simulink model "soc_WLAN_fpga"  (R2024b)
settings: Solver=FixedStepDiscrete  StartTime=0.0  StopTime=stopTime  RelTol=1e-3
PreLoadFcn:
  | addpath(fullfile(matlabroot,'toolbox','whdl','whdlexamples','whdlexamples'));
InitFcn:
  | addpath(fullfile(matlabroot,'toolbox','whdl','whdlexamples','whdlexamples'));
model workspace (MAT data in the model file):
  socvcb : containers.Map (value not decoded)
undefined symbols (not defined in the file): Add, bitRatePerOfdmSym, chanBW, coe, cpLen, dataUpsampleFactor, DelayValMaxNsdMinusLastPilotSc, DescramblerInitialSeed, designMultirateFIR, fftLen, filterLatency, filterUpsampleFactor, Fs, Hd, HT_MFMCS0, HT_MFMCS1, HT_MFMCS2, HT_MFMCS3, HT_MFMCS4, HT_MFMCS5, HT_MFMCS6, HT_MFMCS7, HTUnUsedScInd, inputSamplingRate, interp_coeff, maxPilotRefCounterVale, maxPilotsRef, maxPilotsRefNonHT, Ncol_HT, Ncol_NonHT, noDataSubCarriers, Non_HTMCS0, Non_HTMCS1, Non_HTMCS2, Non_HTMCS3, Non_HTMCS4, Non_HTMCS5, Non_HTMCS6, Non_HTMCS7, Nrow_HT, Nrow_NonHT, numDSC_HT, numDSC_HT_vhtSigB, numDSC_NonHT, numDscHT, numDscNonHT, numOfBitsPerOFDMSym, numOfDataBitsPerOFDMSym, numPilots, numScHT, numSCS_HT, numSCS_NonHT, pnSeq, QAM, rxDownsampleFactor, secondPIdx_HT, secondPIdx_NonHT, Shift, VHTMCS0, VHTMCS1 ... (+7)
libraries: hdlsllib x267, simulink x210, dspsigops x22, whdlutilities x10, whdlmod x9, dsphdlfiltering2 x5, dsphdlmathfun2 x4, whdledac x3, hwlogicconnlib x2, commhdlcrc x2, dsphdlsigops2 x2
(part 6 of 14)

== system soc_WLAN_fpga/WLAN/WLAN HDL/WLAN_Tx_Rx/WLAN_Rx/WLANHDLReceiver/DataRecovery/Deinterleaver/averageVhtSigBbits ==
  dataIn : Inport
  startIn : Inport  Port=2
  endIn : Inport  Port=3
  validIn : Inport  Port=4
  numSCSFlag : Inport  Port=5
  format : Inport  Port=6
  rst : Inport  Port=7
  Add : Sum
  Compare To Constant : simulink/Logic and Bit Operations/Compare To Constant  relop===  const=2  OutDataTypeStr=boolean
  Compare To Constant1 : simulink/Logic and Bit Operations/Compare To Constant  relop===  const=2  OutDataTypeStr=boolean
  Compare To Constant2 : simulink/Logic and Bit Operations/Compare To Constant  relop=<=  const=numDSC_HT-1  OutDataTypeStr=boolean
  Constant : Constant  Value=chanBW  OutDataTypeStr=fixdt(0,3,0)  SampleTime=-1
  Delay1 : Delay  DelayLength=54
  Delay2 : Delay  DelayLength=54
  Delay3 : Delay  DelayLength=54
  HDL Counter : hdlsllib/Sources/HDL Counter  CountType=Count limited  CountInit=0  CountStep=1  CountMax=65535  CountFromType=Initial value  CountFrom=0  CountResetPort=on  CountLoadPort=off  CountEnbPort=on  CountDirPort=off  CountHitOutputPort=off  CountDataType=Unsigned  CountWordLen=16  CountFracLen=0  CountSampTime=1
  Logical Operator : Logic  Inputs=4  AllPortsSameDT=off  OutDataTypeStr=boolean
  Logical Operator1 : Logic  AllPortsSameDT=off  OutDataTypeStr=boolean
  Shift Arithmetic : ArithShift  BitShiftNumber=1  BitShiftDirection=Right
  Switch : Switch  Criteria=u2 ~= 0  SaturateOnIntegerOverflow=off  InputSameDT=off
  Switch1 : Switch  Criteria=u2 ~= 0  SaturateOnIntegerOverflow=off  InputSameDT=off
  Switch2 : Switch  Criteria=u2 ~= 0  SaturateOnIntegerOverflow=off  InputSameDT=off
  dataOut : Outport
  startOut : Outport  Port=2
  endOut : Outport  Port=3
  validOut : Outport  Port=4
  wires:
  Constant/1 -> Compare To Constant/1
  Add/1 -> Shift Arithmetic/1
  numSCSFlag/1 -> Logical Operator/2
  dataIn/1 -> Add/1, Delay3/1, Switch/3
  Delay3/1 -> Add/2
  Compare To Constant/1 -> Logical Operator/1
  validIn/1 -> HDL Counter/2, Switch1/3, Delay1/1, Logical Operator1/2
  Delay1/1 -> Logical Operator1/1
  Logical Operator1/1 -> Switch1/1
  Logical Operator/1 -> Switch/2, Switch2/2, Switch1/2
  Switch1/1 -> validOut/1
  startIn/1 -> Switch2/3, Delay2/1
  Delay2/1 -> Switch2/1
  Switch2/1 -> startOut/1
  endIn/1 -> endOut/1
  Switch/1 -> dataOut/1
  Shift Arithmetic/1 -> Switch/1
  format/1 -> Compare To Constant1/1
  Compare To Constant1/1 -> Logical Operator/3
  HDL Counter/1 -> Compare To Constant2/1
  Compare To Constant2/1 -> Logical Operator/4
  rst/1 -> HDL Counter/1

== system soc_WLAN_fpga/WLAN/WLAN HDL/WLAN_Tx_Rx/WLAN_Rx/WLANHDLReceiver/FrameFormatDetectionAndSignalRecovery/CRCCheckAndBitInterpretation/numOFDMSymbolCalVHT ==
  note: Compute the number of OFDM data symbols for VHT frame format
  PSDULenNonHT : Inport
  numSTS : Inport  Port=2
  1-D Lookup Table : Lookup_n-D  NumberOfTableDimensions=1  BreakpointsForDimension1=[1:8]  IndexSearchMethod=Evenly spaced points  Table=9+[1 2 4 4 6 6 8 8]  ExtrapMethod=Clip  UseLastTableValue=on  InternalRulePriority=Speed  RndMeth=Simplest
  Add : Sum  Inputs=+-  OutDataTypeStr=uint16
  Delay : Delay  DelayLength=1
  Delay1 : Delay  DelayLength=1
  Delay2 : Delay  DelayLength=1
  Shift Arithmetic : ArithShift  BitShiftNumber=2  BitShiftDirection=Right
  rxTimeVHT : Subsystem
  numOFDMSymbVHT : Outport
  wires:
  numSTS/1 -> 1-D Lookup Table/1
  Shift Arithmetic/1 -> Delay/1
  1-D Lookup Table/1 -> Delay1/1
  Add/1 -> Delay2/1
  PSDULenNonHT/1 -> rxTimeVHT/1(In1)
  rxTimeVHT/1(Out1) -> Shift Arithmetic/1
  Delay/1 -> Add/1
  Delay1/1 -> Add/2
  Delay2/1 -> numOFDMSymbVHT/1

== system soc_WLAN_fpga/WLAN/WLAN HDL/WLAN_Tx_Rx/WLAN_Rx/WLANHDLReceiver/FrameFormatDetectionAndSignalRecovery/FormatIdentification/isQBPSK ==
  note: Threshold chose as half of used subcarriers in signal fields
  dataIn : Inport
  validIn : Inport  Port=2
  symbCount : Inport  Port=3
  rst : Inport  Port=4
  Compare To Constant : simulink/Logic and Bit Operations/Compare To Constant  relop===  const=5  OutDataTypeStr=boolean
  Compare To Constant1 : simulink/Logic and Bit Operations/Compare To Constant  relop===  const=6  OutDataTypeStr=boolean
  Complex to Real-Imag : ComplexToRealImag
  Constant : Constant  Value=48*0.5  OutDataTypeStr=fixdt(0,5,0)  SampleTime=-1
  Delay : Delay
  Delay1 : Delay
  Delay2 : Delay  DelayLength=1
  Delay3 : Delay  DelayLength=1
  Delay4 : Delay  DelayLength=3
  Delay5 : Delay  DelayLength=3
  Delay6 : Delay  DelayLength=3
  HDL Counter1 : hdlsllib/Sources/HDL Counter  CountType=Count limited  CountInit=0  CountStep=1  CountMax=256  CountFromType=Initial value  CountFrom=0  CountResetPort=on  CountLoadPort=off  CountEnbPort=on  CountDirPort=off  CountHitOutputPort=off  CountDataType=Unsigned  CountWordLen=9  CountFracLen=0  CountSampTime=1
  Logical Operator : Logic  AllPortsSameDT=off  OutDataTypeStr=boolean
  Logical Operator1 : Logic  AllPortsSameDT=off  OutDataTypeStr=boolean
  Logical Operator2 : Logic  Operator=OR  AllPortsSameDT=off  OutDataTypeStr=boolean
  Product : Product
  Product1 : Product
  Relational Operator : RelationalOperator  Operator=>  OutDataTypeStr=boolean  RndMeth=Simplest  InputSameDT=off
  Relational Operator1 : RelationalOperator  Operator=>  OutDataTypeStr=boolean  RndMeth=Simplest  InputSameDT=off
  To Workspace : ToWorkspace  VariableName=formatData  SampleTime=-1
      settings: Save2DSignal=2-D array (concatenate along first dimension)
  To Workspace1 : ToWorkspace  VariableName=formatValid  SampleTime=-1
      settings: Save2DSignal=2-D array (concatenate along first dimension)
  isQBPSK : Outport
  wires:
  Product/1 -> Delay2/1
  Complex to Real-Imag/2 -> Delay1/1
  Complex to Real-Imag/1 -> Delay/1
  Product1/1 -> Delay3/1
  dataIn/1 -> Delay5/1, Complex to Real-Imag/1
  HDL Counter1/1 -> Relational Operator1/1
  Constant/1 -> Relational Operator1/2
  Relational Operator1/1 -> isQBPSK/1
  Delay/1 -> Product/2, Product/1
  Delay1/1 -> Product1/2, Product1/1
  Delay2/1 -> Relational Operator/2
  Delay3/1 -> Relational Operator/1
  Relational Operator/1 -> Logical Operator/1
  Logical Operator/1 -> HDL Counter1/2
  validIn/1 -> Delay4/1
  Delay4/1 -> Logical Operator1/1
  symbCount/1 -> Compare To Constant1/1, Compare To Constant/1
  Compare To Constant/1 -> Logical Operator2/1
  Logical Operator1/1 -> Logical Operator/2, To Workspace1/1
  Delay6/1 -> Logical Operator1/2
  Compare To Constant1/1 -> Logical Operator2/2
  Logical Operator2/1 -> Delay6/1
  rst/1 -> HDL Counter1/1
  Delay5/1 -> To Workspace/1

== system soc_WLAN_fpga/WLAN/WLAN HDL/WLAN_Tx_Rx/WLAN_Rx/WLANHDLReceiver/FrameFormatDetectionAndSignalRecovery/SignalBitRecovery/Deinterleaver Block ==
  note: Give null output if valid is LOW
  dataIn : Inport
  startIn : Inport  Port=2
  endIn : Inport  Port=3
  validIn : Inport  Port=4
  Constant : Constant  Value=0  OutDataTypeStr=Inherit: Inherit via back propagation  SampleTime=-1
  Delay{1,3..6,9..11} (8 alike) : Delay  DelayLength=1
  Delay12 : Delay  DelayLength=7
  Delay13 : Delay  DelayLength=7
  Delay14 : Delay  DelayLength=7
  Delay{2,15..17} (4 alike) : Delay
  Delay7 : Delay  DelayLength=1  InitialCondition=true
  Delay8 : Delay  DelayLength=1  InitialCondition=true
  Generate Ready : Subsystem
  Logical Operator : Logic  IconShape=distinctive  AllPortsSameDT=off  OutDataTypeStr=boolean
  RAM : hdlsllib/HDL RAMs/Simple Dual Port RAM  ram_size=nextpow2(2*maxBlkSize)
  Read Logic : Subsystem
  Store Block Lengths : hdlsllib/HDL RAMs/HDL FIFO  fifo_size=4  mode=Classic  ratio=1  push_msg=Warning  pop_msg=Ignore  show_empty=off  show_full=off  show_num=on  LabelModeActiveChoice_Mode=Classic  rst_port=off
  Switch : Switch  Criteria=u2 ~= 0  SaturateOnIntegerOverflow=off
  Write Logic : Subsystem
  dataOut : Outport
  startOut : Outport  Port=2
  endOut : Outport  Port=3
  validOut : Outport  Port=4
  ready : Outport  Port=5
  wires:
  Delay17/1 -> Delay14/1
  Delay16/1 -> Delay12/1
  Delay15/1 -> Delay13/1
  Delay14/1 -> RAM/1
  Delay12/1 -> RAM/2
  Delay13/1 -> RAM/3
  Constant/1 -> Switch/3
  Switch/1 -> dataOut/1
  RAM/1 -> Switch/1
  Generate Ready/1(ready) -> ready/1, [ready]
  Read Logic/6(advPop) -> Generate Ready/1(advPop)
  Write Logic/5(endReady) -> Generate Ready/4(endReady)
  Delay7/1 -> Logical Operator/2
  validIn/1 -> Logical Operator/1
  Logical Operator/1 -> Write Logic/2(valid)
  [ready] -> Delay7/1
  Read Logic/5(pop) -> [b]
  Delay6/1 -> startOut/1
  Delay10/1 -> validOut/1, Switch/2
  Delay5/1 -> endOut/1
  Delay11/1 -> Store Block Lengths/2
  Delay9/1 -> Store Block Lengths/1
  Delay4/1 -> Delay15/1
  Delay3/1 -> Delay16/1
  Delay1/1 -> Delay17/1
  Delay8/1 -> Store Block Lengths/3, Generate Ready/3(pop)
  [b] -> Delay8/1
  Read Logic/3(end) -> Delay5/1
  Read Logic/2(start) -> Delay6/1
  Read Logic/1(rdAddr) -> RAM/4
  Store Block Lengths/1 -> Read Logic/1(fifoData)
  Read Logic/4(valid) -> Delay10/1
  Write Logic/4(endOut) -> Delay11/1
  Write Logic/3(count) -> Delay9/1
  Write Logic/2(wrValid) -> Delay4/1
  Write Logic/1(wrAddr) -> Delay3/1
  endIn/1 -> Write Logic/3(end)
  startIn/1 -> Write Logic/1(start)
  Delay2/1 -> Delay1/1
  dataIn/1 -> Delay2/1
  Store Block Lengths/2 -> Read Logic/2(fifoCount), Generate Ready/2(fifoCount)

== system soc_WLAN_fpga/WLAN/WLAN HDL/WLAN_Tx_Rx/WLAN_Rx/WLANHDLReceiver/FrameFormatDetectionAndSignalRecovery/SignalBitRecovery/ViterbiDecoder ==
  llr : Inport
  ctrlIn : Inport  Port=2
  Gain : Gain  Gain=-1  OutDataTypeStr=Inherit: Same as input
  Viterbi Decoder : whdledac/Viterbi Decoder  ConstraintLength=7  CodeGenerator=[133 171]  ErasureInputPort=off  Tbd=32  TerminationMethod=Truncated  ResetInputPort=off  SimulateUsing=Code generation
  bit : Outport
  ctrlOut : Outport  Port=2
  wires:
  Viterbi Decoder/1 -> bit/1
  Viterbi Decoder/2 -> ctrlOut/1
  ctrlIn/1 -> Viterbi Decoder/2
  llr/1 -> Gain/1
  Gain/1 -> Viterbi Decoder/1

== system soc_WLAN_fpga/WLAN/WLAN HDL/WLAN_Tx_Rx/WLAN_Rx/WLANHDLReceiver/FrameFormatDetectionAndSignalRecovery/averageSigFieldsFor40MHz/averager ==
  In1 : Inport
  enb : Inport  Port=2
  rst : Inport  Port=3
  Add : Sum
  Compare To Constant : simulink/Logic and Bit Operations/Compare To Constant  relop=>=  const=numDSC_NonHT/2  OutDataTypeStr=boolean
  Constant : Constant  Value=complex(0,0)  OutDataTypeStr=Inherit: Inherit via back propagation  SampleTime=-1
  Delay : Delay  DelayLength=fftLen/2
  Gain : Gain  Gain=0.5
  HDL Counter : hdlsllib/Sources/HDL Counter  CountType=Count limited  CountInit=0  CountStep=1  CountMax=numDSC_NonHT-1  CountFromType=Initial value  CountFrom=0  CountResetPort=on  CountLoadPort=off  CountEnbPort=on  CountDirPort=off  CountHitOutputPort=off  CountDataType=Unsigned  CountWordLen=8  CountFracLen=0  CountSampTime=1
  Logical Operator : Logic  AllPortsSameDT=off  OutDataTypeStr=boolean
  Switch : Switch  Criteria=u2 ~= 0  SaturateOnIntegerOverflow=off  InputSameDT=off
  Out1 : Outport
  validIn : Outport  Port=2
  wires:
  Constant/1 -> Switch/3
  In1/1 -> Delay/1, Add/1
  HDL Counter/1 -> Compare To Constant/1
  Delay/1 -> Add/2
  Compare To Constant/1 -> Logical Operator/1, Switch/2
  Add/1 -> Gain/1
  enb/1 -> Logical Operator/2, HDL Counter/2
  Switch/1 -> Out1/1
  Gain/1 -> Switch/1
  Logical Operator/1 -> validIn/1
  rst/1 -> HDL Counter/1

== system soc_WLAN_fpga/WLAN/WLAN HDL/WLAN_Tx_Rx/WLAN_Rx/WLANHDLReceiver/HT_VHTCPEEstAndCorrection/CPECorrector/Reciprocal ==
  dataIn : Inport
  Compare To Constant : simulink/Logic and Bit Operations/Compare To Constant  relop=<  const=0  OutDataTypeStr=boolean
  Data Type Conversion : DataTypeConversion  OutDataTypeStr=fixdt(1,WL,0)  ConvertRealWorld=Stored Integer (SI)  SaturateOnIntegerOverflow=off  RndMeth=Floor
  Data Type Conversion1 : DataTypeConversion  OutDataTypeStr=fixdt(0,LUTAddrWL,0)  ConvertRealWorld=Stored Integer (SI)  SaturateOnIntegerOverflow=off  RndMeth=Floor
  Data Type Conversion2 : DataTypeConversion  OutDataTypeStr=fixdt(0,WL-LUTAddrWL,0)  ConvertRealWorld=Stored Integer (SI)  SaturateOnIntegerOverflow=off  RndMeth=Floor
  Delay : Delay  DelayLength=1
  Delay1 : Delay  DelayLength=1
  Delay2 : Delay  DelayLength=1
  Extract Bits : simulink/Logic and Bit Operations/Extract Bits  bitsToExtract=Range ending with least significant bit  numBits=LUTAddrWL  bitIdxRange=[0 7]  outScalingMode=Treat bit field as an integer
  Function Impl : Subsystem
  dataOut : Outport
  wires:
  Data Type Conversion2/1 -> Function Impl/1(switch)
  Delay2/1 -> Data Type Conversion1/1
  Delay1/1 -> Data Type Conversion2/1
  Delay/1 -> Extract Bits/1, Compare To Constant/1
  Function Impl/1(functionValues) -> dataOut/1
  Data Type Conversion1/1 -> Function Impl/2(LUTAddr)
  Compare To Constant/1 -> Delay1/1
  Data Type Conversion/1 -> Delay/1
  Extract Bits/1 -> Delay2/1
  dataIn/1 -> Data Type Conversion/1

== system soc_WLAN_fpga/WLAN/WLAN HDL/WLAN_Tx_Rx/WLAN_Rx/WLANHDLReceiver/HT_VHTCPEEstAndCorrection/CPEEstimator/RefrenceSignalGen ==
  note: reference pilots are stored in LUT for 4 symbols
      | pilots for 4 symbols are stored to avoid modulo operation
  note: Counter for pilot Subcarriers for 4 Symbols
  loadIn : Inport
  vhtSigB : Inport  Port=2
  rst : Inport  Port=3
  1-D Lookup Table1 : Lookup_n-D  NumberOfTableDimensions=1  BreakpointsForDimension1=[0:maxPilotsRef^2-1]  IndexSearchMethod=Evenly spaced points  Table=PilotsDataDec.'  ExtrapMethod=Clip  UseLastTableValue=on  InternalRulePriority=Speed  OutDataTypeStr=fixdt(1,2,0)  RndMeth=Simplest
  Compare To Constant : simulink/Logic and Bit Operations/Compare To Constant  relop===  const=numSCS_HT-1  OutDataTypeStr=boolean
  Delay : Delay  DelayLength=1  InitialCondition=0  UseCircularBuffer=on
  HDL Counter : hdlsllib/Sources/HDL Counter  CountType=Count limited  CountInit=0  CountStep=1  CountMax=maxPilotsRef^2-1  CountFromType=Initial value  CountFrom=0  CountResetPort=on  CountLoadPort=off  CountEnbPort=on  CountDirPort=off  CountHitOutputPort=off  CountDataType=Unsigned  CountWordLen=maxPilotRefCounterVale*2  CountFracLen=0  CountSampTime=1
  HDL Counter1 : hdlsllib/Sources/HDL Counter  CountType=Count limited  CountInit=0  CountStep=1  CountMax=numSCS_HT-1  CountFromType=Initial value  CountFrom=0  CountResetPort=on  CountLoadPort=off  CountEnbPort=on  CountDirPort=off  CountHitOutputPort=off  CountDataType=Unsigned  CountWordLen=8  CountFracLen=0  CountSampTime=1
  Logical Operator : Logic  AllPortsSameDT=off  OutDataTypeStr=boolean
  Logical Operator1 : Logic  Operator=OR  AllPortsSameDT=off  OutDataTypeStr=boolean
  RefPilotsOut : Outport
  wires:
  HDL Counter/1 -> 1-D Lookup Table1/1
  1-D Lookup Table1/1 -> Delay/1
  loadIn/1 -> HDL Counter/2
  vhtSigB/1 -> Logical Operator/2, HDL Counter1/2
  HDL Counter1/1 -> Compare To Constant/1
  Compare To Constant/1 -> Logical Operator/1
  Logical Operator/1 -> Logical Operator1/1
  rst/1 -> Logical Operator1/2, HDL Counter1/1
  Logical Operator1/1 -> HDL Counter/1
  Delay/1 -> RefPilotsOut/1

== system soc_WLAN_fpga/WLAN/WLAN HDL/WLAN_Tx_Rx/WLAN_Rx/WLANHDLReceiver/HT_VHTChannelEstAndEqualize/ChannelEqualizer/validForEqualization ==
  note: selecting Data field for equalization
  validIn : Inport
  symbNum : Inport  Port=2
  rst : Inport  Port=3
  Compare To Constant1 : simulink/Logic and Bit Operations/Compare To Constant  relop=>=  const=9  OutDataTypeStr=boolean
  Compare To Constant2 : simulink/Logic and Bit Operations/Compare To Constant  relop===  const=9  OutDataTypeStr=boolean
  Compare To Constant3 : simulink/Logic and Bit Operations/Compare To Constant  relop===  const=0  OutDataTypeStr=boolean
  HDL Counter : hdlsllib/Sources/HDL Counter  CountType=Count limited  CountInit=0  CountStep=1  CountMax=numSCS_HT-1  CountFromType=Initial value  CountFrom=0  CountResetPort=on  CountLoadPort=off  CountEnbPort=on  CountDirPort=off  CountHitOutputPort=off  CountDataType=Unsigned  CountWordLen=8  CountFracLen=0  CountSampTime=1
  Logical Operator : Logic  AllPortsSameDT=off  OutDataTypeStr=boolean
  Logical Operator1 : Logic  AllPortsSameDT=off  OutDataTypeStr=boolean
  Logical Operator2 : Logic  AllPortsSameDT=off  OutDataTypeStr=boolean
  hValid : Outport
  DataValid : Outport  Port=2
  loadH : Outport  Port=3
  wires:
  validIn/1 -> Logical Operator1/1, Logical Operator/1
  Logical Operator/1 -> DataValid/1
  symbNum/1 -> Compare To Constant2/1, Compare To Constant1/1
  Compare To Constant1/1 -> Logical Operator/2
  Compare To Constant2/1 -> Logical Operator1/2
  Logical Operator2/1 -> loadH/1
  HDL Counter/1 -> Compare To Constant3/1
  Logical Operator1/1 -> Logical Operator2/2, HDL Counter/2, hValid/1
  Compare To Constant3/1 -> Logical Operator2/1
  rst/1 -> HDL Counter/1

== system soc_WLAN_fpga/WLAN/WLAN HDL/WLAN_Tx_Rx/WLAN_Rx/WLANHDLReceiver/NonHTCPEEstAndCorrection/CPECorrector/Reciprocal ==
  dataIn : Inport
  Compare To Constant : simulink/Logic and Bit Operations/Compare To Constant  relop=<  const=0  OutDataTypeStr=boolean
  Data Type Conversion : DataTypeConversion  OutDataTypeStr=fixdt(1,WL,0)  ConvertRealWorld=Stored Integer (SI)  SaturateOnIntegerOverflow=off  RndMeth=Floor
  Data Type Conversion1 : DataTypeConversion  OutDataTypeStr=fixdt(0,LUTAddrWL,0)  ConvertRealWorld=Stored Integer (SI)  SaturateOnIntegerOverflow=off  RndMeth=Floor
  Data Type Conversion2 : DataTypeConversion  OutDataTypeStr=fixdt(0,WL-LUTAddrWL,0)  ConvertRealWorld=Stored Integer (SI)  SaturateOnIntegerOverflow=off  RndMeth=Floor
  Delay : Delay  DelayLength=1
  Delay1 : Delay  DelayLength=1
  Delay2 : Delay  DelayLength=1
  Extract Bits : simulink/Logic and Bit Operations/Extract Bits  bitsToExtract=Range ending with least significant bit  numBits=LUTAddrWL  bitIdxRange=[0 7]  outScalingMode=Treat bit field as an integer
  Function Impl : Subsystem
  dataOut : Outport
  wires:
  Data Type Conversion2/1 -> Function Impl/1(switch)
  Delay2/1 -> Data Type Conversion1/1
  Delay1/1 -> Data Type Conversion2/1
  Delay/1 -> Extract Bits/1, Compare To Constant/1
  Function Impl/1(functionValues) -> dataOut/1
  Data Type Conversion1/1 -> Function Impl/2(LUTAddr)
  Compare To Constant/1 -> Delay1/1
  Data Type Conversion/1 -> Delay/1
  Extract Bits/1 -> Delay2/1
  dataIn/1 -> Data Type Conversion/1

== system soc_WLAN_fpga/WLAN/WLAN HDL/WLAN_Tx_Rx/WLAN_Rx/WLANHDLReceiver/NonHTCPEEstAndCorrection/CPEEstimator/RefrenceSignalGen ==
  note: reference pilots are stored in LUT for 4 symbols
      | pilots for 4 symbols are stored to avoid modulo operation
  note: Counter for pilot Subcarriers for 4 Symbols
  loadIn : Inport
  rst : Inport  Port=2
  1-D Lookup Table1 : Lookup_n-D  NumberOfTableDimensions=1  BreakpointsForDimension1=[0:maxPilotsRefNonHT-1]  IndexSearchMethod=Evenly spaced points  Table=PilotLUTSignalNonHT.'  TableDataTypeStr=fixdt(1,2,0)  ExtrapMethod=Clip  UseLastTableValue=on  InternalRulePriority=Speed  OutDataTypeStr=fixdt(1,2,0)  RndMeth=Simplest
  Delay2 : Delay  DelayLength=1  InitialCondition=0  UseCircularBuffer=on
  HDL Counter : hdlsllib/Sources/HDL Counter  CountType=Count limited  CountInit=0  CountStep=1  CountMax=maxPilotsRefNonHT-1  CountFromType=Initial value  CountFrom=0  CountResetPort=on  CountLoadPort=off  CountEnbPort=on  CountDirPort=off  CountHitOutputPort=off  CountDataType=Unsigned  CountWordLen=3  CountFracLen=0  CountSampTime=1
  RefPilotsOut : Outport
  wires:
  HDL Counter/1 -> 1-D Lookup Table1/1
  1-D Lookup Table1/1 -> Delay2/1
  loadIn/1 -> HDL Counter/2
  rst/1 -> HDL Counter/1
  Delay2/1 -> RefPilotsOut/1

== system soc_WLAN_fpga/WLAN/WLAN HDL/WLAN_Tx_Rx/WLAN_Rx/WLANHDLReceiver/NonHTChannelEstAndEqualize/ChannelEqualizer/NonHTDataSelector ==
  note: selecting from L-SIG field to L-Data for equalization
  validIn : Inport
  symbNum : Inport  Port=2
  Compare To Constant1 : simulink/Logic and Bit Operations/Compare To Constant  relop=>=  const=4  OutDataTypeStr=boolean
  Logical Operator : Logic  AllPortsSameDT=off  OutDataTypeStr=boolean
  NonHTValid : Outport
  wires:
  validIn/1 -> Logical Operator/2
  Logical Operator/1 -> NonHTValid/1
  symbNum/1 -> Compare To Constant1/1
  Compare To Constant1/1 -> Logical Operator/1

== system soc_WLAN_fpga/WLAN/WLAN HDL/WLAN_Tx_Rx/WLAN_Rx/WLANHDLReceiver/OFDMDemodulation/Symbol Counter/vhtRotation ==
  u : Inport
  In2 : Inport  Port=2
  Compare To Constant : simulink/Logic and Bit Operations/Compare To Constant  relop=>=  const=fftLen/2  OutDataTypeStr=boolean
  Constant : Constant  Value=fi(1/1i,1,2,0)  SampleTime=-1
  Product : Product
  Switch : Switch  Criteria=u2 ~= 0  SaturateOnIntegerOverflow=off  InputSameDT=off
  dataOut : Outport
  wires:
  In2/1 -> Switch/3, Product/1
  Constant/1 -> Product/2
  Switch/1 -> dataOut/1
  Compare To Constant/1 -> Switch/2
  u/1 -> Compare To Constant/1
  Product/1 -> Switch/1

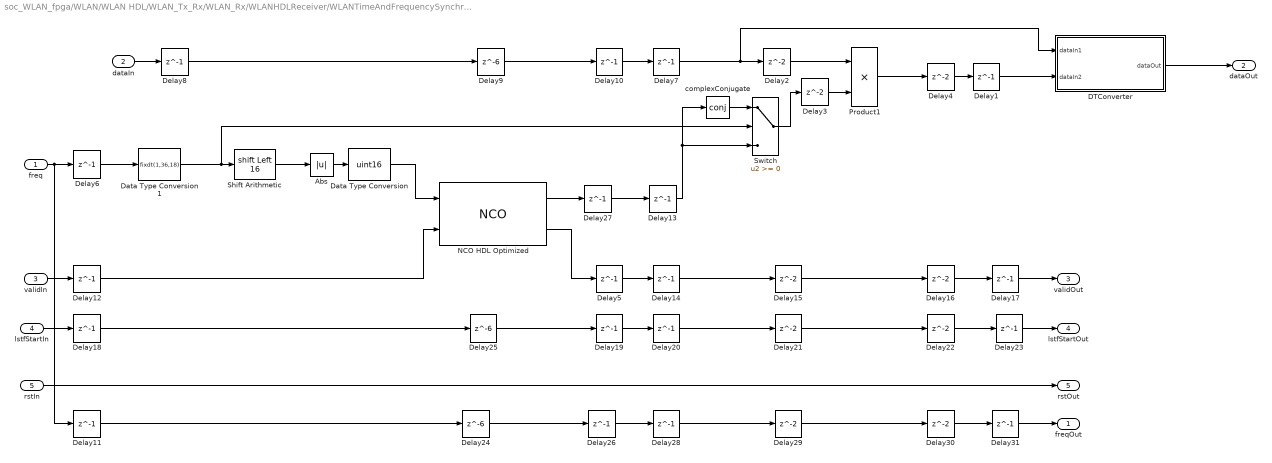
== system soc_WLAN_fpga/WLAN/WLAN HDL/WLAN_Tx_Rx/WLAN_Rx/WLANHDLReceiver/WLANTimeAndFrequencySynchronization/Coarse CFO Estimation and Correction/Coarse CFO Correction ==
  freq : Inport
  dataIn : Inport  Port=2
  validIn : Inport  Port=3
  lstfStartIn : Inport  Port=4
  rstIn : Inport  Port=5
  Abs : Abs  SaturateOnIntegerOverflow=off
  DTConverter : MATLAB Function  TreatAsAtomicUnit=on
  Data Type Conversion : DataTypeConversion  OutDataTypeStr=uint16  RndMeth=Round  SaturateOnIntegerOverflow=off
  Data Type Conversion1 : DataTypeConversion  OutDataTypeStr=fixdt(1,36,18)  SaturateOnIntegerOverflow=off  RndMeth=Floor
  Delay{1,5..8,10..14,17..20,23,26..28,31} (19 alike) : Delay  DelayLength=1  InitialCondition=0  UseCircularBuffer=on
  Delay{2..4,15..16,21..22,29..30} (9 alike) : Delay  InitialCondition=0  UseCircularBuffer=on
  Delay24 : Delay  DelayLength=6  InitialCondition=0  UseCircularBuffer=on
  Delay25 : Delay  DelayLength=6  InitialCondition=0  UseCircularBuffer=on
  Delay9 : Delay  DelayLength=6  InitialCondition=0  UseCircularBuffer=on
  NCO HDL Optimized : dsphdlsigops2/NCO  PhaseIncrementSource=Input port  PhaseIncrement=100  PhaseOffsetSource=Property  PhaseOffset=0  DitherSource=None  NumDitherBits=4  SamplesPerFrame=1  LUTCompress=off  ResetAction=off  Waveform=Complex exponential  PhasePort=off  SimulateUsing=Code generation  AccumulatorWL=16  PhaseQuantization=on  NumQuantizerAccumulatorBits=16  OutputDataType=Binary point scaling  OutputWL=16  OutputFL=14
  Product1 : Product
  Shift Arithmetic : ArithShift  BitShiftNumber=16  BitShiftDirection=Left
  Switch : Switch  SaturateOnIntegerOverflow=off  InputSameDT=off
  complexConjugate : Math  Operator=conj  SignedPower=on
  freqOut : Outport  VectorParamsAs1DForOutWhenUnconnected=off
  dataOut : Outport  Port=2  VectorParamsAs1DForOutWhenUnconnected=off
  validOut : Outport  Port=3  VectorParamsAs1DForOutWhenUnconnected=off
  lstfStartOut : Outport  Port=4  VectorParamsAs1DForOutWhenUnconnected=off
  rstOut : Outport  Port=5  VectorParamsAs1DForOutWhenUnconnected=off
  wires:
  Delay25/1 -> Delay19/1
  NCO HDL Optimized/2 -> Delay5/1
  Delay9/1 -> Delay10/1
  Delay23/1 -> lstfStartOut/1
  Delay22/1 -> Delay23/1
  Delay21/1 -> Delay22/1
  Delay20/1 -> Delay21/1
  Delay19/1 -> Delay20/1
  Delay18/1 -> Delay25/1
  lstfStartIn/1 -> Delay18/1
  Delay5/1 -> Delay14/1
  freq/1 -> Delay11/1, Delay6/1
  Delay4/1 -> Delay1/1
  dataIn/1 -> Delay8/1
  Delay17/1 -> validOut/1
  Delay3/1 -> Product1/2
  Delay16/1 -> Delay17/1
  validIn/1 -> Delay12/1
  Delay10/1 -> Delay7/1
  Delay15/1 -> Delay16/1
  Delay2/1 -> Product1/1
  Product1/1 -> Delay4/1
  Delay13/1 -> complexConjugate/1, Switch/3
  Delay8/1 -> Delay9/1
  Delay7/1 -> DTConverter/1(dataIn1), Delay2/1
  Delay14/1 -> Delay15/1
  Delay27/1 -> Delay13/1
  Data Type Conversion/1 -> NCO HDL Optimized/1
  Delay12/1 -> NCO HDL Optimized/2
  NCO HDL Optimized/1 -> Delay27/1
  rstIn/1 -> rstOut/1
  Delay6/1 -> Data Type Conversion1/1
  Data Type Conversion1/1 -> Shift Arithmetic/1, Switch/2
  DTConverter/1(dataOut) -> dataOut/1
  Delay1/1 -> DTConverter/2(dataIn2)
  complexConjugate/1 -> Switch/1
  Switch/1 -> Delay3/1
  Shift Arithmetic/1 -> Abs/1
  Abs/1 -> Data Type Conversion/1
  Delay11/1 -> Delay24/1
  Delay24/1 -> Delay26/1
  Delay26/1 -> Delay28/1
  Delay28/1 -> Delay29/1
  Delay29/1 -> Delay30/1
  Delay30/1 -> Delay31/1
  Delay31/1 -> freqOut/1

== system soc_WLAN_fpga/WLAN/WLAN HDL/WLAN_Tx_Rx/WLAN_Rx/WLANHDLReceiver/WLANTimeAndFrequencySynchronization/Coarse CFO Estimation and Correction/Coarse CFO Estimation ==
  dataIn : Inport
  validIn : Inport  Port=2
  LSTF_start : Inport  Port=3
  rstIn : Inport  Port=4
  Complex to Magnitude-Angle HDL Optimized : dsphdlmathfun2/Complex to Magnitude-Angle  NumIterationsSource=Auto  NumIterations=30  OutputFormat=Angle  AngleFormat=Normalized  ScaleOutput=off  ScalingMethod=Shift-Add  SimulateUsing=Code generation
  Delay10 : Delay  DelayLength=wlanConfig.lstfLen  InitialCondition=0
  Delay{11,13,16..17,21} (5 alike) : Delay  DelayLength=1  InitialCondition=0  UseCircularBuffer=on
  Delay14 : Delay  DelayLength=wlanConfig.lstfLen  InitialCondition=0
  Delay15 : Delay  InitialCondition=0  UseCircularBuffer=on
  Delay22 : Delay  DelayLength=35  InitialCondition=0  UseCircularBuffer=on
  Delay23 : Delay  DelayLength=round(wlanConfig.lstfLen*0.75)+8*wlanConfig.lstfLen-1  InitialCondition=0  UseCircularBuffer=on
  Delay{24..27} (4 alike) : Delay  DelayLength=1
  Delay4 : Delay  DelayLength=35  InitialCondition=0  UseCircularBuffer=on
  Delay5 : Delay  DelayLength=35  InitialCondition=0  UseCircularBuffer=on
  Delay6 : Delay  InitialCondition=0  UseCircularBuffer=on
  Delay7 : Delay  DelayLength=round(wlanConfig.lstfLen*0.75)+8*wlanConfig.lstfLen-1  InitialCondition=0  UseCircularBuffer=on
  Delay9 : Delay  DelayLength=round(wlanConfig.lstfLen*0.75)+8*wlanConfig.lstfLen-1  InitialCondition=0  UseCircularBuffer=on
  Shift Arithmetic : ArithShift  BitShiftNumber=log2(2*wlanConfig.lstfLen)  BitShiftDirection=Right
  Unit Delay Enabled Resettable Synchronous : hdlsllib/Discrete/Unit Delay Enabled Resettable Synchronous  InitialCondition=0.0  SampleTime=-1
  averager : Subsystem
  correlator : Subsystem
  Freq : Outport  VectorParamsAs1DForOutWhenUnconnected=off
  dataOut : Outport  Port=2  VectorParamsAs1DForOutWhenUnconnected=off
  validData : Outport  Port=3  VectorParamsAs1DForOutWhenUnconnected=off
  lstfStart : Outport  Port=4  VectorParamsAs1DForOutWhenUnconnected=off
  rstOut : Outport  Port=5  VectorParamsAs1DForOutWhenUnconnected=off
  wires:
  validIn/1 -> Delay10/1
  dataIn/1 -> Delay14/1, correlator/1(dataIn)
  LSTF_start/1 -> correlator/2(lstf_start)
  Delay9/1 -> Delay5/1
  Complex to Magnitude-Angle HDL Optimized/2 -> Delay13/1
  Delay5/1 -> Delay16/1
  Delay4/1 -> Delay17/1
  Complex to Magnitude-Angle HDL Optimized/1 -> Delay11/1
  Delay16/1 -> validData/1
  Delay17/1 -> dataOut/1
  Delay10/1 -> Delay6/1
  Delay6/1 -> Delay26/1
  Delay11/1 -> Shift Arithmetic/1
  Delay7/1 -> Delay4/1
  Delay26/1 -> Delay9/1
  Delay14/1 -> Delay15/1
  Delay15/1 -> Delay27/1
  Delay27/1 -> Delay7/1
  Delay22/1 -> Delay21/1
  correlator/2(load) -> Delay25/1
  Delay23/1 -> Delay22/1
  Delay21/1 -> lstfStart/1
  Delay25/1 -> Delay23/1, averager/2(load)
  Shift Arithmetic/1 -> Unit Delay Enabled Resettable Synchronous/1
  Unit Delay Enabled Resettable Synchronous/1 -> Freq/1
  Delay13/1 -> Unit Delay Enabled Resettable Synchronous/2
  rstIn/1 -> averager/3(rst), Unit Delay Enabled Resettable Synchronous/3, rstOut/1
  correlator/1(corrOut) -> Delay24/1
  averager/1(avgCorr) -> Complex to Magnitude-Angle HDL Optimized/1
  averager/2(validOut) -> Complex to Magnitude-Angle HDL Optimized/2
  Delay24/1 -> averager/1(corrIn)

== system soc_WLAN_fpga/WLAN/WLAN HDL/WLAN_Tx_Rx/WLAN_Rx/WLANHDLReceiver/WLANTimeAndFrequencySynchronization/Coarse Time Sync/correlator ==
  dataIn : Inport
  validIn : Inport  Port=2
  startIn : Inport  Port=3
  Constant : Constant  Value=complex(0,0)  VectorParams1D=off  OutDataTypeStr=Inherit: Inherit via back propagation  SampleTime=-1
  Delay : Delay
  Delay1 : Delay  DelayLength=1
  Delay2 : Delay  DelayLength=wlanConfig.lstfLen-1
  Delay3 : Delay
  Delay4 : Delay  DelayLength=1
  Delay5 : Delay  DelayLength=1
  Logical Operator : Logic  AllPortsSameDT=off  OutDataTypeStr=boolean
  MagnitudeSquared : Subsystem
  MovingSum : Subsystem  InitFcn=Simulink.suppressDiagnostic(gcb, 'SimulinkFixedPoint:util:Overflowoccurred');
  Shift Arithmetic : ArithShift  BitShiftNumber=log2(wlanConfig.lstfLen)  BitShiftDirection=Right
  Switch : Switch  Criteria=u2 > Threshold  SaturateOnIntegerOverflow=off  InputSameDT=off
  delayedCorrelation : Subsystem
  dataOut : Outport
  validOut : Outport  Port=2
  wires:
  MagnitudeSquared/2(validOut) -> Delay3/1
  MovingSum/2(validOut) -> Delay2/1, Logical Operator/2
  Switch/1 -> Shift Arithmetic/1
  Constant/1 -> Switch/3
  MovingSum/1(dataOut) -> Switch/1
  Logical Operator/1 -> MagnitudeSquared/2(validIn), Switch/2
  Delay2/1 -> Logical Operator/1
  MagnitudeSquared/1(dataOut) -> Delay/1
  Shift Arithmetic/1 -> MagnitudeSquared/1(dataIn)
  Delay/1 -> dataOut/1
  Delay3/1 -> validOut/1
  dataIn/1 -> delayedCorrelation/1(dataIn)
  validIn/1 -> delayedCorrelation/2(validIn)
  startIn/1 -> delayedCorrelation/3(startIn)
  delayedCorrelation/1(corrOut) -> Delay1/1
  delayedCorrelation/2(corrValid) -> Delay4/1
  delayedCorrelation/3(startOut) -> Delay5/1
  Delay1/1 -> MovingSum/1(dataIn)
  Delay4/1 -> MovingSum/2(validIn)
  Delay5/1 -> MovingSum/3(reset)

== system soc_WLAN_fpga/WLAN/WLAN HDL/WLAN_Tx_Rx/WLAN_Rx/WLANHDLReceiver/WLANTimeAndFrequencySynchronization/Coarse Time Sync/energyCalculator ==
  corrIn : Inport
  corrValidIn : Inport  Port=2
  dataIn : Inport  Port=3
  validIn : Inport  Port=4
  Delay : Delay  DelayLength=1
  Delay1 : Delay
  Delay2 : Delay
  Enabled Delay : Delay  DelayLength=1  ShowEnablePort=on
      settings: InputPortMap=u0,e6
  Enabled Delay1 : Delay  DelayLength=1  ShowEnablePort=on
      settings: InputPortMap=u0,e6
  magnitudeSquared : Subsystem
  corrOut : Outport
  energyOut : Outport  Port=2
  validOut : Outport  Port=3
  wires:
  validIn/1 -> magnitudeSquared/2(validIn)
  Enabled Delay/1 -> energyOut/1
  magnitudeSquared/1(energy) -> Delay1/1
  corrValidIn/1 -> Enabled Delay/2, Enabled Delay1/2
  Enabled Delay1/1 -> validOut/1
  magnitudeSquared/2(push) -> Delay2/1
  dataIn/1 -> magnitudeSquared/1(dataIn)
  corrIn/1 -> Delay/1
  Delay/1 -> corrOut/1
  Delay1/1 -> Enabled Delay/1
  Delay2/1 -> Enabled Delay1/1

== system soc_WLAN_fpga/WLAN/WLAN HDL/WLAN_Tx_Rx/WLAN_Rx/WLANHDLReceiver/WLANTimeAndFrequencySynchronization/Coarse Time Sync/peakDetection ==
  note: Searching peak in LSTF region
  corrIn : Inport
  energyIn : Inport  Port=2
  corrValid : Inport  Port=3
  dataIn : Inport  Port=4
  dataValid : Inport  Port=5
  Delay1 : Delay  DelayLength=wlanConfig.lstfLen*10  InitialCondition=0  UseCircularBuffer=on
  Delay2 : Delay  DelayLength=wlanConfig.lstfLen*10  InitialCondition=0  UseCircularBuffer=on
  Logical Operator3 : Logic  AllPortsSameDT=off  OutDataTypeStr=boolean
  MATLAB Function1 : MATLAB Function  TreatAsAtomicUnit=on
  Relational Operator : RelationalOperator  Operator=>  OutDataTypeStr=boolean  InputSameDT=off
  considerFirstPeak : Subsystem
  searchStartOfFrame : MATLAB Function  TreatAsAtomicUnit=on
  lstfStart : Outport
  validOut : Outport  Port=2
  dataOut : Outport  Port=3
  wires:
  Relational Operator/1 -> searchStartOfFrame/1(thresholdValid)
  Logical Operator3/1 -> validOut/1, MATLAB Function1/1(syncEn)
  energyIn/1 -> Relational Operator/2
  dataValid/1 -> Delay1/1
  corrValid/1 -> searchStartOfFrame/2(valid)
  dataIn/1 -> Delay2/1
  Delay2/1 -> MATLAB Function1/2(dataIn)
  MATLAB Function1/1(dataOut) -> dataOut/1
  searchStartOfFrame/1(syncOut) -> considerFirstPeak/1(peakIn)
  considerFirstPeak/1(peakOut) -> lstfStart/1
  considerFirstPeak/2(validOut) -> Logical Operator3/1
  corrIn/1 -> Relational Operator/1
  Delay1/1 -> MATLAB Function1/3(validIn), Logical Operator3/2

== system soc_WLAN_fpga/WLAN/WLAN HDL/WLAN_Tx_Rx/WLAN_Rx/WLANHDLReceiver/WLANTimeAndFrequencySynchronization/Coarse Time Sync/streamSynchrnizer ==
  corrValid : Inport
  dataIn : Inport  Port=2
  dataValid : Inport  Port=3
  Delay5 : Delay  DelayLength=wlanConfig.lstfLen-1
  Enabled Delay : Delay  DelayLength=1  ShowEnablePort=on
      settings: InputPortMap=u0,e6
  Enabled Delay1 : Delay  DelayLength=1  ShowEnablePort=on
      settings: InputPortMap=u0,e6
  Logical Operator8 : Logic  Operator=OR  AllPortsSameDT=off  OutDataTypeStr=boolean
  dataOut : Outport
  validOut : Outport  Port=2
  wires:
  Enabled Delay1/1 -> validOut/1
  corrValid/1 -> Logical Operator8/2, Delay5/1
  Delay5/1 -> Logical Operator8/1
  dataValid/1 -> Enabled Delay1/1
  dataIn/1 -> Enabled Delay/1
  Logical Operator8/1 -> Enabled Delay/2, Enabled Delay1/2
  Enabled Delay/1 -> dataOut/1

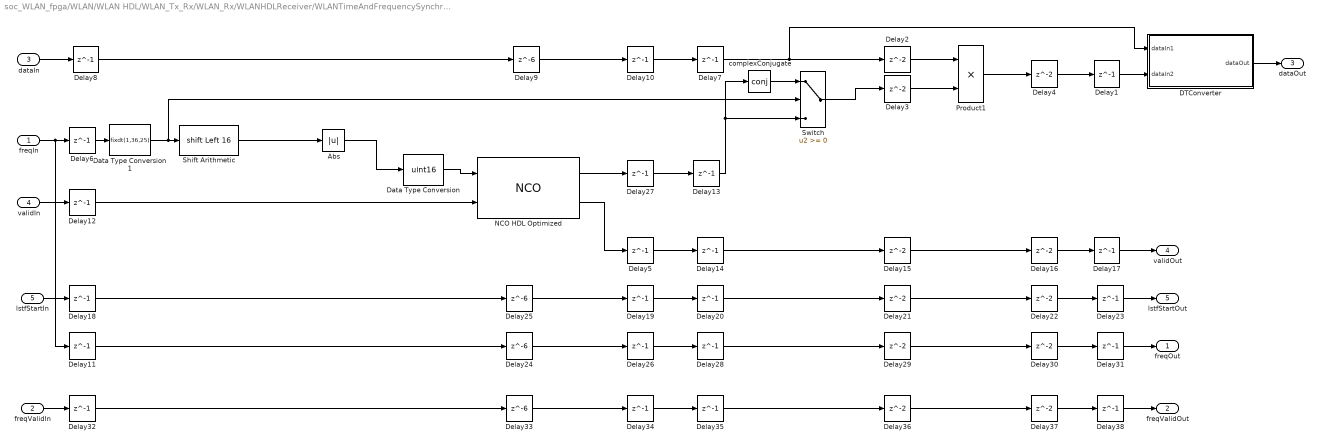
== system soc_WLAN_fpga/WLAN/WLAN HDL/WLAN_Tx_Rx/WLAN_Rx/WLANHDLReceiver/WLANTimeAndFrequencySynchronization/Fine CFO Estimation and Correction/Fine CFO Correction ==
  freqIn : Inport
  freqValidIn : Inport  Port=2
  dataIn : Inport  Port=3
  validIn : Inport  Port=4
  lstfStartIn : Inport  Port=5
  Abs : Abs  SaturateOnIntegerOverflow=off
  DTConverter : MATLAB Function  TreatAsAtomicUnit=on
  Data Type Conversion : DataTypeConversion  OutDataTypeStr=uint16  SaturateOnIntegerOverflow=off  RndMeth=Floor
  Data Type Conversion1 : DataTypeConversion  OutDataTypeStr=fixdt(1,36,25)  SaturateOnIntegerOverflow=off  RndMeth=Floor
  Delay{1,5..8,10..14,17..20,23,26..28,31..32,34..35,38} (23 alike) : Delay  DelayLength=1  InitialCondition=0  UseCircularBuffer=on
  Delay{2..4,15..16,21..22,29..30,36..37} (11 alike) : Delay  InitialCondition=0  UseCircularBuffer=on
  Delay{9,24..25,33} (4 alike) : Delay  DelayLength=6  InitialCondition=0  UseCircularBuffer=on
  NCO HDL Optimized : dsphdlsigops2/NCO  PhaseIncrementSource=Input port  PhaseIncrement=100  PhaseOffsetSource=Property  PhaseOffset=0  DitherSource=None  NumDitherBits=4  SamplesPerFrame=1  LUTCompress=off  ResetAction=off  Waveform=Complex exponential  PhasePort=off  SimulateUsing=Code generation  AccumulatorWL=16  PhaseQuantization=on  NumQuantizerAccumulatorBits=16  OutputDataType=Binary point scaling  OutputWL=16  OutputFL=12
  Product1 : Product
  Shift Arithmetic : ArithShift  BitShiftNumber=16  BitShiftDirection=Left
  Switch : Switch  SaturateOnIntegerOverflow=off  InputSameDT=off
  complexConjugate : Math  Operator=conj  SignedPower=on
  freqOut : Outport  VectorParamsAs1DForOutWhenUnconnected=off
  freqValidOut : Outport  Port=2  VectorParamsAs1DForOutWhenUnconnected=off
  dataOut : Outport  Port=3  VectorParamsAs1DForOutWhenUnconnected=off
  validOut : Outport  Port=4  VectorParamsAs1DForOutWhenUnconnected=off
  lstfStartOut : Outport  Port=5  VectorParamsAs1DForOutWhenUnconnected=off
  wires:
  Delay25/1 -> Delay19/1
  NCO HDL Optimized/2 -> Delay5/1
  Delay9/1 -> Delay10/1
  Delay23/1 -> lstfStartOut/1
  Delay22/1 -> Delay23/1
  Delay21/1 -> Delay22/1
  Delay20/1 -> Delay21/1
  Delay19/1 -> Delay20/1
  Delay18/1 -> Delay25/1
  lstfStartIn/1 -> Delay18/1
  Delay5/1 -> Delay14/1
  freqIn/1 -> Delay11/1, Delay6/1
  Delay4/1 -> Delay1/1
  dataIn/1 -> Delay8/1
  Delay17/1 -> validOut/1
  Delay3/1 -> Product1/2
  Delay16/1 -> Delay17/1
  validIn/1 -> Delay12/1
  Delay10/1 -> Delay7/1
  Delay15/1 -> Delay16/1
  Delay2/1 -> Product1/1
  Product1/1 -> Delay4/1
  Delay13/1 -> Switch/3, complexConjugate/1
  Delay8/1 -> Delay9/1
  Delay7/1 -> DTConverter/1(dataIn1), Delay2/1
  Delay14/1 -> Delay15/1
  Delay27/1 -> Delay13/1
  Data Type Conversion/1 -> NCO HDL Optimized/1
  Delay12/1 -> NCO HDL Optimized/2
  NCO HDL Optimized/1 -> Delay27/1
  Delay6/1 -> Data Type Conversion1/1
  Data Type Conversion1/1 -> Switch/2, Shift Arithmetic/1
  DTConverter/1(dataOut) -> dataOut/1
  Delay1/1 -> DTConverter/2(dataIn2)
  Switch/1 -> Delay3/1
  complexConjugate/1 -> Switch/1
  Shift Arithmetic/1 -> Abs/1
  Delay11/1 -> Delay24/1
  Delay24/1 -> Delay26/1
  Delay26/1 -> Delay28/1
  Delay28/1 -> Delay29/1
  Delay29/1 -> Delay30/1
  Delay30/1 -> Delay31/1
  Delay31/1 -> freqOut/1
  freqValidIn/1 -> Delay32/1
  Delay32/1 -> Delay33/1
  Delay33/1 -> Delay34/1
  Delay34/1 -> Delay35/1
  Delay35/1 -> Delay36/1
  Delay36/1 -> Delay37/1
  Delay37/1 -> Delay38/1
  Delay38/1 -> freqValidOut/1
  Abs/1 -> Data Type Conversion/1

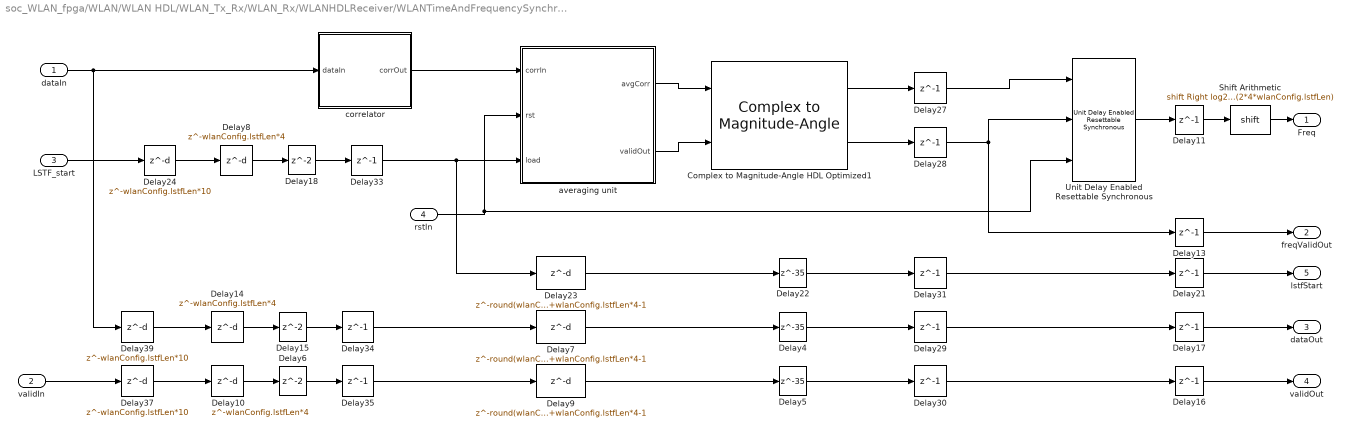
== system soc_WLAN_fpga/WLAN/WLAN HDL/WLAN_Tx_Rx/WLAN_Rx/WLANHDLReceiver/WLANTimeAndFrequencySynchronization/Fine CFO Estimation and Correction/Fine CFO Estimation ==
  dataIn : Inport
  validIn : Inport  Port=2
  LSTF_start : Inport  Port=3
  rstIn : Inport  Port=4
  Complex to Magnitude-Angle HDL Optimized1 : dsphdlmathfun2/Complex to Magnitude-Angle  NumIterationsSource=Auto  NumIterations=30  OutputFormat=Angle  AngleFormat=Normalized  ScaleOutput=off  ScalingMethod=Shift-Add  SimulateUsing=Code generation
  Delay10 : Delay  DelayLength=wlanConfig.lstfLen*4  InitialCondition=0
  Delay{11,13,16..17,21} (5 alike) : Delay  DelayLength=1  InitialCondition=0  UseCircularBuffer=on
  Delay14 : Delay  DelayLength=wlanConfig.lstfLen*4  InitialCondition=0
  Delay15 : Delay  InitialCondition=0  UseCircularBuffer=on
  Delay18 : Delay  InitialCondition=0  UseCircularBuffer=on
  Delay22 : Delay  DelayLength=35  InitialCondition=0  UseCircularBuffer=on
  Delay23 : Delay  DelayLength=round(wlanConfig.lstfLen*2*0.75)+wlanConfig.lstfLen*4-1  InitialCondition=0  UseCircularBuffer=on
  Delay24 : Delay  DelayLength=wlanConfig.lstfLen*10  InitialCondition=0
  Delay{27..31,33..35} (8 alike) : Delay  DelayLength=1
  Delay37 : Delay  DelayLength=wlanConfig.lstfLen*10  InitialCondition=0
  Delay39 : Delay  DelayLength=wlanConfig.lstfLen*10  InitialCondition=0
  Delay4 : Delay  DelayLength=35  InitialCondition=0  UseCircularBuffer=on
  Delay5 : Delay  DelayLength=35  InitialCondition=0  UseCircularBuffer=on
  Delay6 : Delay  InitialCondition=0  UseCircularBuffer=on
  Delay7 : Delay  DelayLength=round(wlanConfig.lstfLen*2*0.75)+wlanConfig.lstfLen*4-1  InitialCondition=0  UseCircularBuffer=on
  Delay8 : Delay  DelayLength=wlanConfig.lstfLen*4  InitialCondition=0
  Delay9 : Delay  DelayLength=round(wlanConfig.lstfLen*2*0.75)+wlanConfig.lstfLen*4-1  InitialCondition=0  UseCircularBuffer=on
  Shift Arithmetic : ArithShift  BitShiftNumber=log2(2*4*wlanConfig.lstfLen)  BitShiftDirection=Right
  Unit Delay Enabled Resettable Synchronous : hdlsllib/Discrete/Unit Delay Enabled Resettable Synchronous  InitialCondition=0.0  SampleTime=-1
  averaging unit : Subsystem
  correlator : Subsystem
  Freq : Outport  VectorParamsAs1DForOutWhenUnconnected=off
  freqValidOut : Outport  Port=2  VectorParamsAs1DForOutWhenUnconnected=off
  dataOut : Outport  Port=3  VectorParamsAs1DForOutWhenUnconnected=off
  validOut : Outport  Port=4  VectorParamsAs1DForOutWhenUnconnected=off
  lstfStart : Outport  Port=5  VectorParamsAs1DForOutWhenUnconnected=off
  wires:
  Delay9/1 -> Delay5/1
  Complex to Magnitude-Angle HDL Optimized1/2 -> Delay28/1
  Complex to Magnitude-Angle HDL Optimized1/1 -> Delay27/1
  Delay5/1 -> Delay30/1
  Delay4/1 -> Delay29/1
  Unit Delay Enabled Resettable Synchronous/1 -> Delay11/1
  Delay13/1 -> freqValidOut/1
  Delay16/1 -> validOut/1
  Delay17/1 -> dataOut/1
  Delay10/1 -> Delay6/1
  Delay8/1 -> Delay18/1
  Delay6/1 -> Delay35/1
  Delay11/1 -> Shift Arithmetic/1
  Shift Arithmetic/1 -> Freq/1
  Delay7/1 -> Delay4/1
  Delay35/1 -> Delay9/1
  Delay14/1 -> Delay15/1
  Delay15/1 -> Delay34/1
  Delay34/1 -> Delay7/1
  Delay22/1 -> Delay31/1
  Delay23/1 -> Delay22/1
  Delay21/1 -> lstfStart/1
  Delay33/1 -> averaging unit/3(load), Delay23/1
  Delay24/1 -> Delay8/1
  LSTF_start/1 -> Delay24/1
  Delay18/1 -> Delay33/1
  Delay27/1 -> Unit Delay Enabled Resettable Synchronous/1
  Delay28/1 -> Unit Delay Enabled Resettable Synchronous/2, Delay13/1
  Delay29/1 -> Delay17/1
  Delay30/1 -> Delay16/1
  Delay31/1 -> Delay21/1
  Delay37/1 -> Delay10/1
  Delay39/1 -> Delay14/1
  validIn/1 -> Delay37/1
  rstIn/1 -> Unit Delay Enabled Resettable Synchronous/3, averaging unit/2(rst)
  dataIn/1 -> correlator/1(dataIn), Delay39/1
  correlator/1(corrOut) -> averaging unit/1(corrIn)
  averaging unit/1(avgCorr) -> Complex to Magnitude-Angle HDL Optimized1/1
  averaging unit/2(validOut) -> Complex to Magnitude-Angle HDL Optimized1/2

== system soc_WLAN_fpga/WLAN/WLAN HDL/WLAN_Tx_Rx/WLAN_Rx/WLANHDLReceiver/WLANTimeAndFrequencySynchronization/Fine Time Sync/correlator ==
  dataIn : Inport
  validIn : Inport  Port=2
  startIn : Inport  Port=3
  rstIn : Inport  Port=4
  Delay : Delay  DelayLength=ceil((filterLatency+filterUpsampleFactor-1)/filterUpsampleFactor - 1)
  Delay1 : Delay  DelayLength=ceil((filterLatency+filterUpsampleFactor-1)/filterUpsampleFactor)
  Delay13 : Delay  DelayLength=3
  Delay15 : Delay  DelayLength=3
  Delay16 : Delay  DelayLength=3
  Delay2 : Delay  DelayLength=ceil((filterLatency+filterUpsampleFactor-1)/filterUpsampleFactor)
  Delay{22..26} (5 alike) : Delay  DelayLength=1
  MagnitudeSquared : Subsystem
  corrFilter : Subsystem
  corrOut : Outport
  corrValid : Outport  Port=2
  startOut : Outport  Port=3
  dataOut : Outport  Port=4
  validOut : Outport  Port=5
  wires:
  corrFilter/1(dataOut) -> Delay22/1
  Delay13/1 -> startOut/1
  startIn/1 -> Delay/1
  Delay22/1 -> MagnitudeSquared/1(dataIn)
  Delay24/1 -> Delay13/1
  Delay/1 -> Delay24/1
  Delay23/1 -> MagnitudeSquared/2(validIn)
  MagnitudeSquared/1(dataOut) -> corrOut/1
  corrFilter/2(validOut) -> Delay23/1
  MagnitudeSquared/2(validOut) -> corrValid/1
  Delay15/1 -> dataOut/1
  Delay16/1 -> validOut/1
  validIn/1 -> Delay2/1, corrFilter/2(validIn)
  dataIn/1 -> corrFilter/1(dataIn), Delay1/1
  Delay1/1 -> Delay25/1
  Delay2/1 -> Delay26/1
  Delay26/1 -> Delay16/1
  Delay25/1 -> Delay15/1
  rstIn/1 -> corrFilter/3(rst)

== system soc_WLAN_fpga/WLAN/WLAN HDL/WLAN_Tx_Rx/WLAN_Rx/WLANHDLReceiver/WLANTimeAndFrequencySynchronization/Fine Time Sync/peakSearcher ==
  corrIn : Inport
  corrValid : Inport  Port=2
  startIn : Inport  Port=3
  dataIn : Inport  Port=4
  validIn : Inport  Port=5
  rstIn : Inport  Port=6
  maxPeakSearcher : Subsystem
  peakDetector : Subsystem
  lstfStart : Outport
  validOut : Outport  Port=2
  dataOut : Outport  Port=3
  wires:
  validIn/1 -> maxPeakSearcher/4(validIn)
  corrIn/1 -> maxPeakSearcher/1(corrIn)
  corrValid/1 -> maxPeakSearcher/2(corrValid)
  startIn/1 -> maxPeakSearcher/3(startIn)
  dataIn/1 -> maxPeakSearcher/5(dataIn)
  maxPeakSearcher/1(maxPeakValue) -> peakDetector/1(maxPeakVal)
  maxPeakSearcher/2(countRst) -> peakDetector/2(counterRst)
  maxPeakSearcher/3(dataOut) -> peakDetector/3(dataIn)
  maxPeakSearcher/4(validOut) -> peakDetector/4(validIn)
  peakDetector/1(lstfStart) -> lstfStart/1
  peakDetector/2(validOut) -> validOut/1
  peakDetector/3(dataOut) -> dataOut/1
  rstIn/1 -> maxPeakSearcher/6(rstIn)

== system soc_WLAN_fpga/WLAN/WLAN HDL/WLAN_Tx_Rx/WLAN_Rx/WLANHDLReceiver/DataRecovery/Decoder/Depuncturer/Depuncturer1 ==
  dataIn : Inport
  rstIn : Inport  Port=2
  startIn : Inport  Port=3
  endIn : Inport  Port=4
  validIn : Inport  Port=5
  Delay : Delay  DelayLength=5
  Delay1 : Delay  DelayLength=5
  Delay{2..3,5..10,15} (9 alike) : Delay  DelayLength=1
  Delay4 : Delay
  Logical Operator4 : Logic  AllPortsSameDT=off  OutDataTypeStr=boolean
  Logical Operator8 : Logic  AllPortsSameDT=off  OutDataTypeStr=boolean
  Logical Operator9 : Logic  AllPortsSameDT=off  OutDataTypeStr=boolean
  Sample Control Bus Creator2 : whdlutilities/Sample Control Bus Creator
  sampleParallel1 : MATLAB Function  TreatAsAtomicUnit=on
  dataOut : Outport
  validOut : Outport  Port=2
  wires:
  dataIn/1 -> Delay7/1
  Delay1/1 -> validOut/1
  Delay/1 -> dataOut/1
  validIn/1 -> Delay10/1
  startIn/1 -> Delay4/1
  endIn/1 -> Delay9/1
  Sample Control Bus Creator2/1 -> Delay1/1
  Logical Operator9/1 -> Sample Control Bus Creator2/3
  Logical Operator4/1 -> Sample Control Bus Creator2/1
  sampleParallel1/3(enb) -> Delay6/1
  Delay8/1 -> Logical Operator4/2
  sampleParallel1/2(validOut) -> Delay5/1
  Logical Operator8/1 -> Sample Control Bus Creator2/2
  sampleParallel1/1(dataOut) -> Delay2/1
  Delay4/1 -> sampleParallel1/2(startIn), Delay8/1
  Delay7/1 -> sampleParallel1/1(dataIn)
  Delay15/1 -> Logical Operator8/2
  Delay5/1 -> Logical Operator9/2
  Delay6/1 -> Logical Operator8/1, Logical Operator9/1, Logical Operator4/1
  rstIn/1 -> Delay3/1
  Delay10/1 -> sampleParallel1/4(validIn)
  Delay2/1 -> Delay/1
  Delay9/1 -> Delay15/1, sampleParallel1/3(endIn)
  Delay3/1 -> sampleParallel1/5(reset)

== system soc_WLAN_fpga/WLAN/WLAN HDL/WLAN_Tx_Rx/WLAN_Rx/WLANHDLReceiver/DataRecovery/Decoder/Depuncturer/Depuncturer2 ==
  dataIn : Inport
  startIn : Inport  Port=2
  codeRate : Inport  Port=3
  endIn : Inport  Port=4
  validIn : Inport  Port=5
  Data Type Conversion : DataTypeConversion  OutDataTypeStr=boolean  SaturateOnIntegerOverflow=off  RndMeth=Floor
  Delay3 : Delay  DelayLength=5
  Depuncturer : whdledac/Depuncturer  OperationMode=Frame  SpecifyInputs=Input port  PuncturingVector=[1;1;0;1;1;0]  SimulateUsing=Code generation
  Sample Control Bus Creator1 : whdlutilities/Sample Control Bus Creator
  Terminator : Terminator
  puncVecSelector : MATLAB Function  TreatAsAtomicUnit=on
  dataOut : Outport
  validOut : Outport  Port=2
  wires:
  validIn/1 -> Sample Control Bus Creator1/3
  Data Type Conversion/1 -> Depuncturer/2
  puncVecSelector/1(puncVec) -> Data Type Conversion/1
  Sample Control Bus Creator1/1 -> Depuncturer/3
  Depuncturer/3 -> Terminator/1
  codeRate/1 -> Delay3/1
  Depuncturer/2 -> validOut/1
  Delay3/1 -> puncVecSelector/2(codeRate)
  dataIn/1 -> Depuncturer/1
  endIn/1 -> Sample Control Bus Creator1/2
  startIn/1 -> Sample Control Bus Creator1/1, puncVecSelector/1(start)
  Depuncturer/1 -> dataOut/1
